simulink model "schema"  (R2015a)
settings: Solver=ode45  StartTime=0.0  StopTime=10.0  RelTol=1e-3
settings Model: Creator=David  LastModifiedBy=David

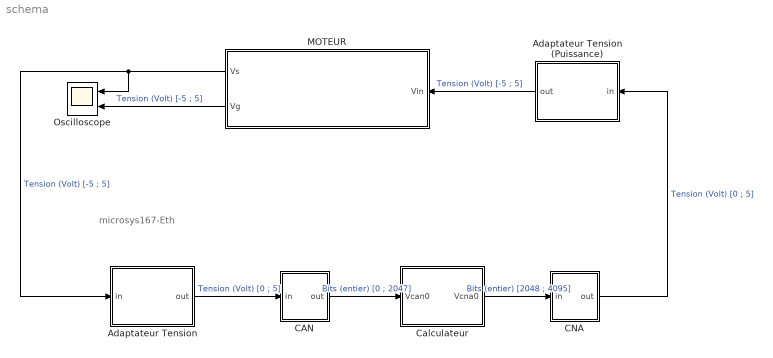
== system schema ==
  note: microsys167-Eth
  Adaptateur Tension : Subsystem
  Adaptateur Tension (Puissance) : Subsystem
  CAN : Subsystem
  CNA : Subsystem
  Calculateur : Subsystem
  MOTEUR : Subsystem
  Oscilloscope : Scope  NumInputPorts=2
      settings: YMin=-5~-5  YMax=5~5
  wires:
  MOTEUR/2(Vg) -> Oscilloscope/2  "Tension (Volt) [-5 ; 5]"
  Adaptateur Tension (Puissance)/1(out) -> MOTEUR/1(Vin)  "Tension (Volt) [-5 ; 5]"
  CNA/1(out) -> Adaptateur Tension (Puissance)/1(in)  "Tension (Volt) [0 ; 5]"
  Calculateur/1(Vcna0) -> CNA/1(in)  "Bits (entier) [2048 ; 4095]"
  CAN/1(out) -> Calculateur/1(Vcan0)  "Bits (entier) [0 ; 2047]"
  Adaptateur Tension/1(out) -> CAN/1(in)  "Tension (Volt) [0 ; 5]"
  MOTEUR/1(Vs) -> Oscilloscope/1, Adaptateur Tension/1(in)  "Tension (Volt) [-5 ; 5]"

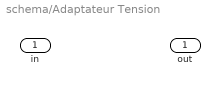
== system schema/Adaptateur Tension ==
  in : Inport
  out : Outport

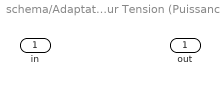
== system schema/Adaptateur Tension (Puissance) ==
  in : Inport
  out : Outport

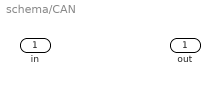
== system schema/CAN ==
  in : Inport
  out : Outport

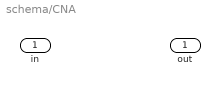
== system schema/CNA ==
  in : Inport
  out : Outport

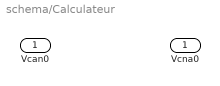
== system schema/Calculateur ==
  Vcan0 : Inport
  Vcna0 : Outport

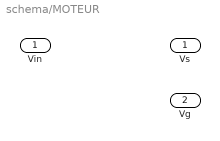
== system schema/MOTEUR ==
  Vin : Inport
  Vs : Outport
  Vg : Outport  Port=2
